simulink model "sampleModel2014"  (R2023a)
settings: Solver=VariableStepAuto  StartTime=0.0  StopTime=10.0  RelTol=1e-3
libraries: hdlsllib x2
settings Model: Creator=user1  LastModifiedBy=user1

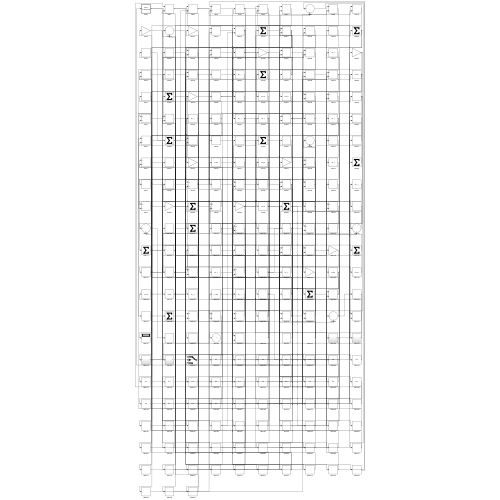
[thumbnail: Simulink's stored preview of the top-level diagram]
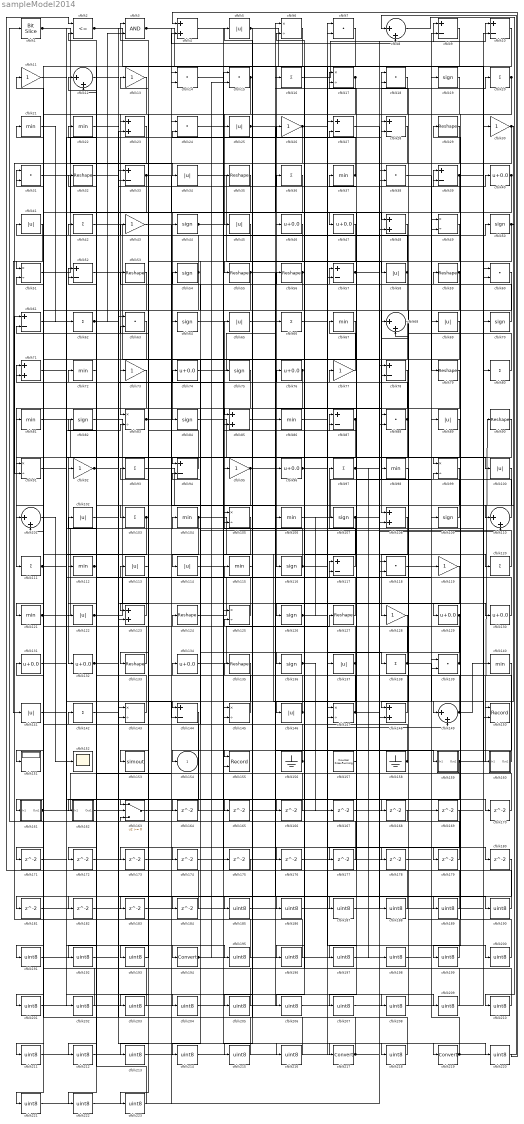
== system sampleModel2014 ==
  cfblk1 : hdlsllib/Logic and Bit Operations/Bit Slice  lidx=7  ridx=0
  cfblk{9..10,27..28,33,39,52,57,61,78,87,94,117,144} (14 alike) : Sum  Inputs=+-
  cfblk{5,25,34,41,45,58,65,69,89,100,102,113..114,122,137,141,146} (17 alike) : Abs  SaturateOnIntegerOverflow=off
  cfblk{8,12,68,101,110,149} (6 alike) : Sum  Inputs=|++
  cfblk{16,20,36,42,62,66,80,93,97,103,111,120,138,142} (14 alike) : Sum  Inputs=+
  cfblk{21..22,37,67,72,81,86,98,104,106,112,115,121,140} (14 alike) : MinMax
  cfblk{6,17,49,51,83,91,99,105,125,143,145,147} (12 alike) : Product  Inputs=*/  RndMeth=Zero  SaturateOnIntegerOverflow=on
  cfblk{19,44,50,54,64,70,75,82,84,107,109,116,126,136} (14 alike) : Signum
  cfblk{4,23,48,71,85,108,123,148} (8 alike) : Sum
  cfblk{11,13,26,30,43,73,77,92,95,119,128} (11 alike) : Gain
  cfblk{7,14..15,18,24,31,38,60,63,88,118,139} (12 alike) : DotProduct  OutDataTypeStr=Inherit: Inherit via internal rule
  cfblk{29,32,35,53,55..56,59,79,90,124,127,133,135} (13 alike) : Reshape
  cfblk{40,46..47,74,76,96,129..132,134} (11 alike) : Bias  Bias=0.0  SaturateOnIntegerOverflow=off
  cfblk150 : Record  FileSettingsInternal="{\"entries\":[{\"content\":{\"excelSettings\":{\"content\":{},\"type\":\"Streamout.ExcelSettings\"}},\"type\":\"Streamout.FileSettingStorage\",\"uuid\":\"\"}],\"packageUris\":[\"http:\\/\\/schema.mathworks.com\\/mf0\\/streamout_blocks\\/R2020a\"],\"version\":\"1.0\"}"  Layout=[1 1]  SignalsInternal="{\"entries\":[{\"content\":{\"signals\":[{\"content\":{\"blockPath\":[],\"dimensions\":[1],\"domain\":\"\",\"lineColor\":\"#a2142f\",\"plots\":[1],\"port\":1,\"signalID\":5947,\"signalName\":\"XY Graph:1\"},\"type\":\"RecordBlkView.Signal\",\"uuid\":\"\"},{\"content\":{\"blockPath\":[],\"dimensions\":[1],\"domain\":\"\",\"lineColor\":\"#139fff\",\"plots\":[1],\"port\":2,\"signalID\":5950,\"signalName\":\"XY Graph:2\"},\"type\":\"RecordBlkView.Signal\",\"uuid\":\"\"}]},\"type\":\"RecordBlkView.InputSignals\",\"uuid\":\"\"}],\"packageUris\":[\"http:\\/\\/schema.mathworks.com\\/mf0\\/streamout_blocks\\/R2020a\"],\"version\":\"1.0\"}"  VisualizationBindings="{\"xyplotplugin\":{\"info\":[{\"series\":[{\"bindingParametersList\":[{\"parameter\":\"X-Axis\",\"signalID\":5947,\"signalName\":\"XY Graph:1\"},{\"parameter\":\"Y-Axis\",\"signalID\":5950,\"signalName\":\"XY Graph:2\"}],\"seriesID\":10914}],\"subplotID\":1}]}}"  CompatibilityTag=XY  st=-1
  cfblk151 : Display
  cfblk152 : Scope
  cfblk153 : ToWorkspace  VariableName=simout  SaveFormat=Timeseries  SampleTime=-1
  cfblk155 : Record  FileSettingsInternal="{\"entries\":[{\"content\":{\"excelSettings\":{\"content\":{},\"type\":\"Streamout.ExcelSettings\"}},\"type\":\"Streamout.FileSettingStorage\",\"uuid\":\"\"}],\"packageUris\":[\"http:\\/\\/schema.mathworks.com\\/mf0\\/streamout_blocks\\/R2020a\"],\"version\":\"1.0\"}"  Layout=[1 1]  SignalsInternal="{\"entries\":[{\"content\":{\"signals\":[{\"content\":{\"blockPath\":[],\"dimensions\":[1],\"domain\":\"\",\"lineColor\":\"#a2142f\",\"plots\":[1],\"port\":1,\"signalID\":5955,\"signalName\":\"XY Graph:1\"},\"type\":\"RecordBlkView.Signal\",\"uuid\":\"\"},{\"content\":{\"blockPath\":[],\"dimensions\":[1],\"domain\":\"\",\"lineColor\":\"#139fff\",\"plots\":[1],\"port\":2,\"signalID\":5958,\"signalName\":\"XY Graph:2\"},\"type\":\"RecordBlkView.Signal\",\"uuid\":\"\"}]},\"type\":\"RecordBlkView.InputSignals\",\"uuid\":\"\"}],\"packageUris\":[\"http:\\/\\/schema.mathworks.com\\/mf0\\/streamout_blocks\\/R2020a\"],\"version\":\"1.0\"}"  VisualizationBindings="{\"xyplotplugin\":{\"info\":[{\"series\":[{\"bindingParametersList\":[{\"parameter\":\"X-Axis\",\"signalID\":5955,\"signalName\":\"XY Graph:1\"},{\"parameter\":\"Y-Axis\",\"signalID\":5958,\"signalName\":\"XY Graph:2\"}],\"seriesID\":54028}],\"subplotID\":1}]}}"  CompatibilityTag=XY  st=-1
  cfblk156 : Ground
  cfblk157 : hdlsllib/Sources/Counter Free-Running  NumBits=16  tsamp=-1
  cfblk158 : Ground
  cfblk159 : Subsystem
      settings: LibrarySourceBlock=|
      | hdlsllib/Ports &
      | Subsystems/Subsystem
  cfblk160 : Subsystem
      settings: LibrarySourceBlock=|
      | hdlsllib/Ports &
      | Subsystems/Subsystem
  cfblk161 : Subsystem
      settings: LibrarySourceBlock=|
      | hdlsllib/Ports &
      | Subsystems/Subsystem
  cfblk162 : Subsystem
      settings: LibrarySourceBlock=|
      | hdlsllib/Ports &
      | Subsystems/Subsystem
  cfblk163 : Switch  SaturateOnIntegerOverflow=off  InputSameDT=off
  cfblk{164..184} (21 alike) : Delay  SampleTime=1
  cfblk{185..193,195..216,218,220..223} (36 alike) : DataTypeConversion  OutDataTypeStr=uint8  SaturateOnIntegerOverflow=off  RndMeth=Floor
  cfblk194 : DataTypeConversion  SaturateOnIntegerOverflow=off  RndMeth=Floor
  cfblk2 : RelationalOperator  Operator=<=  OutDataTypeStr=boolean  InputSameDT=off
  cfblk217 : DataTypeConversion  SaturateOnIntegerOverflow=off  RndMeth=Floor
  cfblk219 : DataTypeConversion  SaturateOnIntegerOverflow=off  RndMeth=Floor
  cfblk3 : Logic  AllPortsSameDT=off  OutDataTypeStr=boolean
  cfblk154 : Outport  VectorParamsAs1DForOutWhenUnconnected=off
  wires:
  cfblk101/1 -> cfblk152/1
  cfblk132/1 -> cfblk75/1, cfblk216/1
  cfblk109/1 -> cfblk18/1
  cfblk21/1 -> cfblk62/1
  cfblk163/1 -> cfblk59/1
  cfblk6/1 -> cfblk116/1
  cfblk159/1(Out1) -> cfblk90/1, cfblk182/1
  cfblk104/1 -> cfblk149/1, cfblk114/1
  cfblk124/1 -> cfblk19/1
  cfblk134/1 -> cfblk127/1
  cfblk116/1 -> cfblk65/1, cfblk138/1
  cfblk30/1 -> cfblk96/1, cfblk110/1
  cfblk82/1 -> cfblk129/1
  cfblk113/1 -> cfblk31/1
  cfblk157/1 -> cfblk37/1
  cfblk89/1 -> cfblk132/1
  cfblk58/1 -> cfblk108/1, cfblk3/1
  cfblk75/1 -> cfblk111/1
  cfblk149/1 -> cfblk87/1, cfblk140/1
  cfblk84/1 -> cfblk99/1
  cfblk34/1 -> cfblk58/1
  cfblk95/1 -> cfblk16/1, cfblk147/2, cfblk192/1
  cfblk98/1 -> cfblk148/1
  cfblk1/1 -> cfblk34/1, cfblk118/2
  cfblk125/1 -> cfblk12/1
  cfblk73/1 -> cfblk121/1
  cfblk54/1 -> cfblk21/1, cfblk81/1
  cfblk29/1 -> cfblk126/1
  cfblk50/1 -> cfblk150/1, cfblk199/1
  cfblk13/1 -> cfblk83/1
  cfblk45/1 -> cfblk163/1
  cfblk143/1 -> cfblk12/2
  cfblk145/1 -> cfblk135/1
  cfblk39/1 -> cfblk80/1, cfblk187/1
  cfblk38/1 -> cfblk79/1
  cfblk4/1 -> cfblk219/1
  cfblk94/1 -> cfblk13/1
  cfblk41/1 -> cfblk141/1
  cfblk51/1 -> cfblk26/1
  cfblk15/1 -> cfblk155/1, cfblk91/1
  cfblk59/1 -> cfblk98/1, cfblk161/1(In1)
  cfblk110/1 -> cfblk77/1
  cfblk103/1 -> cfblk153/1, cfblk201/1
  cfblk146/1 -> cfblk105/1, cfblk124/1
  cfblk25/1 -> cfblk47/1, cfblk20/1
  cfblk97/1 -> cfblk40/1, cfblk198/1
  cfblk96/1 -> cfblk137/1, cfblk180/1
  cfblk133/1 -> cfblk52/1
  cfblk17/1 -> cfblk23/1, cfblk35/1, cfblk143/2
  cfblk108/1 -> cfblk128/1
  cfblk36/1 -> cfblk84/1
  cfblk123/1 -> cfblk22/1
  cfblk20/1 -> cfblk151/1, cfblk189/1
  cfblk87/1 -> cfblk103/1, cfblk211/1
  cfblk147/1 -> cfblk134/1, cfblk117/2, cfblk39/2
  cfblk93/1 -> cfblk105/2
  cfblk16/1 -> cfblk9/1
  cfblk74/1 -> cfblk6/1
  cfblk81/1 -> cfblk94/1
  cfblk79/1 -> cfblk133/1
  cfblk129/1 -> cfblk176/1, cfblk177/1
  cfblk32/1 -> cfblk143/1
  cfblk52/1 -> cfblk73/1
  cfblk64/1 -> cfblk50/1
  cfblk9/1 -> cfblk101/1
  cfblk46/1 -> cfblk55/1
  cfblk42/1 -> cfblk148/2
  cfblk49/1 -> cfblk85/1
  cfblk57/1 -> cfblk10/1, cfblk110/2
  cfblk156/1 -> cfblk113/1, cfblk94/2
  cfblk2/1 -> cfblk95/1, cfblk165/1
  cfblk130/1 -> cfblk76/1
  cfblk121/1 -> cfblk70/1, cfblk83/2
  cfblk26/1 -> cfblk149/2, cfblk91/2
  cfblk61/1 -> cfblk194/1
  cfblk119/1 -> cfblk136/1
  cfblk76/1 -> cfblk112/1, cfblk181/1
  cfblk31/1 -> cfblk44/1
  cfblk138/1 -> cfblk41/1, cfblk150/2
  cfblk92/1 -> cfblk33/1, cfblk36/1
  cfblk142/1 -> cfblk217/1
  cfblk83/1 -> cfblk39/1, cfblk173/1
  cfblk88/1 -> cfblk31/2, cfblk183/1
  cfblk35/1 -> cfblk51/1
  cfblk107/1 -> cfblk179/1, cfblk196/1
  cfblk126/1 -> cfblk107/1, cfblk178/1
  cfblk33/1 -> cfblk48/1, cfblk171/1
  cfblk120/1 -> cfblk54/1
  cfblk18/1 -> cfblk45/1
  cfblk122/1 -> cfblk9/2, cfblk130/1
  cfblk112/1 -> cfblk32/1, cfblk162/1(In1)
  cfblk70/1 -> cfblk57/1
  cfblk43/1 -> cfblk106/1
  cfblk37/1 -> cfblk17/1, cfblk24/2
  cfblk67/1 -> cfblk122/1
  cfblk48/1 -> cfblk86/1
  cfblk111/1 -> cfblk104/1, cfblk144/2
  cfblk127/1 -> cfblk74/1
  cfblk136/1 -> cfblk6/2, cfblk166/1, cfblk167/1
  cfblk47/1 -> cfblk64/1
  cfblk139/1 -> cfblk71/1, cfblk99/2
  cfblk148/1 -> cfblk125/2
  cfblk118/1 -> cfblk89/1
  cfblk3/1 -> cfblk160/1(In1), cfblk8/2
  cfblk140/1 -> cfblk154/1
  cfblk105/1 -> cfblk155/2
  cfblk19/1 -> cfblk123/1
  cfblk55/1 -> cfblk101/2, cfblk88/1
  cfblk161/1(Out1) -> cfblk24/1, cfblk28/1
  cfblk62/1 -> cfblk33/2, cfblk3/2
  cfblk77/1 -> cfblk67/1
  cfblk44/1 -> cfblk28/2, cfblk220/1
  cfblk85/1 -> cfblk159/1(In1)
  cfblk5/1 -> cfblk25/1, cfblk147/1
  cfblk53/1 -> cfblk92/1
  cfblk23/1 -> cfblk123/2
  cfblk117/1 -> cfblk97/1
  cfblk28/1 -> cfblk145/2
  cfblk12/1 -> cfblk120/1
  cfblk106/1 -> cfblk69/1
  cfblk10/1 -> cfblk46/1
  cfblk71/1 -> cfblk100/1
  cfblk40/1 -> cfblk48/2, cfblk203/1
  cfblk131/1 -> cfblk117/1
  cfblk160/1(Out1) -> cfblk93/1
  cfblk114/1 -> cfblk87/2
  cfblk56/1 -> cfblk146/1, cfblk172/1
  cfblk80/1 -> cfblk53/1
  cfblk158/1 -> cfblk17/2, cfblk5/1
  cfblk137/1 -> cfblk144/1, cfblk2/2, cfblk42/1
  cfblk144/1 -> cfblk164/1
  cfblk164/1 -> cfblk71/2
  cfblk165/1 -> cfblk49/2
  cfblk166/1 -> cfblk52/2
  cfblk167/1 -> cfblk10/2
  cfblk91/1 -> cfblk168/1
  cfblk168/1 -> cfblk1/1
  cfblk86/1 -> cfblk170/1
  cfblk170/1 -> cfblk125/1
  cfblk172/1 -> cfblk139/2
  cfblk99/1 -> cfblk174/1
  cfblk174/1 -> cfblk85/2
  cfblk24/1 -> cfblk175/1
  cfblk175/1 -> cfblk2/1
  cfblk176/1 -> cfblk38/1
  cfblk177/1 -> cfblk163/3
  cfblk178/1 -> cfblk18/2
  cfblk179/1 -> cfblk145/1
  cfblk181/1 -> cfblk88/2
  cfblk182/1 -> cfblk108/2
  cfblk183/1 -> cfblk57/2
  cfblk69/1 -> cfblk184/1
  cfblk184/1 -> cfblk43/1
  cfblk60/1 -> cfblk185/1
  cfblk185/1 -> cfblk119/1
  cfblk22/1 -> cfblk186/1
  cfblk186/1 -> cfblk60/1
  cfblk187/1 -> cfblk60/2
  cfblk27/1 -> cfblk188/1
  cfblk188/1 -> cfblk15/1
  cfblk189/1 -> cfblk27/1
  cfblk65/1 -> cfblk190/1
  cfblk190/1 -> cfblk27/2
  cfblk63/1 -> cfblk191/1
  cfblk191/1 -> cfblk23/2
  cfblk192/1 -> cfblk63/1
  cfblk169/1 -> cfblk193/1
  cfblk193/1 -> cfblk63/2
  cfblk194/1 -> cfblk169/1, cfblk15/2
  cfblk141/1 -> cfblk195/1
  cfblk195/1 -> cfblk61/1
  cfblk196/1 -> cfblk61/2
  cfblk68/1 -> cfblk197/1
  cfblk197/1 -> cfblk109/1
  cfblk198/1 -> cfblk68/1
  cfblk199/1 -> cfblk68/2
  cfblk66/1 -> cfblk200/1
  cfblk200/1 -> cfblk29/1
  cfblk201/1 -> cfblk66/1
  cfblk11/1 -> cfblk202/1
  cfblk202/1 -> cfblk51/2
  cfblk203/1 -> cfblk11/1
  cfblk102/1 -> cfblk204/1
  cfblk204/1 -> cfblk30/1
  cfblk100/1 -> cfblk205/1
  cfblk205/1 -> cfblk102/1
  cfblk78/1 -> cfblk206/1
  cfblk206/1 -> cfblk139/1
  cfblk90/1 -> cfblk207/1
  cfblk207/1 -> cfblk78/1
  cfblk171/1 -> cfblk208/1
  cfblk208/1 -> cfblk78/2
  cfblk14/1 -> cfblk209/1
  cfblk209/1 -> cfblk56/1
  cfblk8/1 -> cfblk210/1
  cfblk210/1 -> cfblk14/1
  cfblk211/1 -> cfblk14/2
  cfblk7/1 -> cfblk212/1
  cfblk212/1 -> cfblk38/2
  cfblk173/1 -> cfblk213/1
  cfblk213/1 -> cfblk7/1
  cfblk128/1 -> cfblk214/1
  cfblk214/1 -> cfblk7/2
  cfblk115/1 -> cfblk215/1
  cfblk215/1 -> cfblk82/1
  cfblk216/1 -> cfblk115/1
  cfblk217/1 -> cfblk163/2, cfblk131/1
  cfblk162/1(Out1) -> cfblk218/1
  cfblk218/1 -> cfblk142/1
  cfblk219/1 -> cfblk8/1, cfblk49/1
  cfblk220/1 -> cfblk4/1
  cfblk180/1 -> cfblk221/1
  cfblk221/1 -> cfblk4/2
  cfblk72/1 -> cfblk222/1
  cfblk222/1 -> cfblk118/1
  cfblk135/1 -> cfblk223/1
  cfblk223/1 -> cfblk72/1

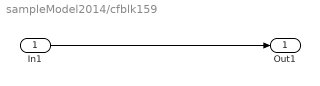
== system sampleModel2014/cfblk159 ==
  In1 : Inport
  Out1 : Outport
  wires:
  In1/1 -> Out1/1

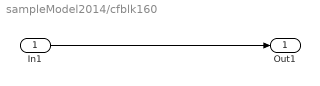
== system sampleModel2014/cfblk160 ==
  In1 : Inport
  Out1 : Outport
  wires:
  In1/1 -> Out1/1

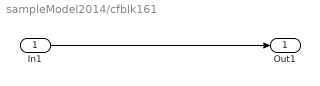
== system sampleModel2014/cfblk161 ==
  In1 : Inport
  Out1 : Outport
  wires:
  In1/1 -> Out1/1

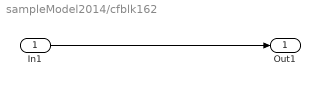
== system sampleModel2014/cfblk162 ==
  In1 : Inport
  Out1 : Outport
  wires:
  In1/1 -> Out1/1
